simulink subsystem "Motores"  (R2023b)
settings: Solver=VariableStepAuto  StartTime=0.0  StopTime=10.0  RelTol=1e-3
libraries: arduinolib x6, simulink x2
settings Model: Creator=mmgac  LastModifiedBy=jaime
settings OptimizationCC: ReuseModelBlockBuffer=off

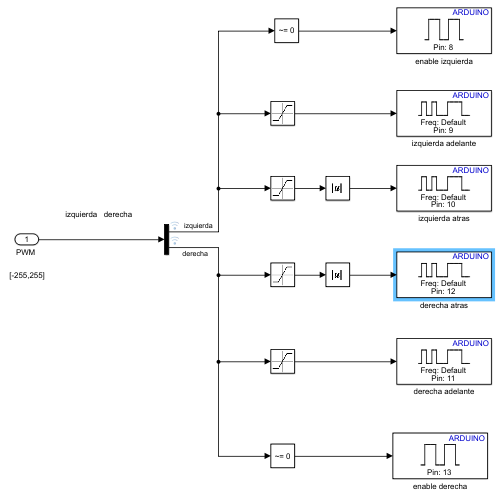
[thumbnail: Simulink's stored preview of the top-level diagram]
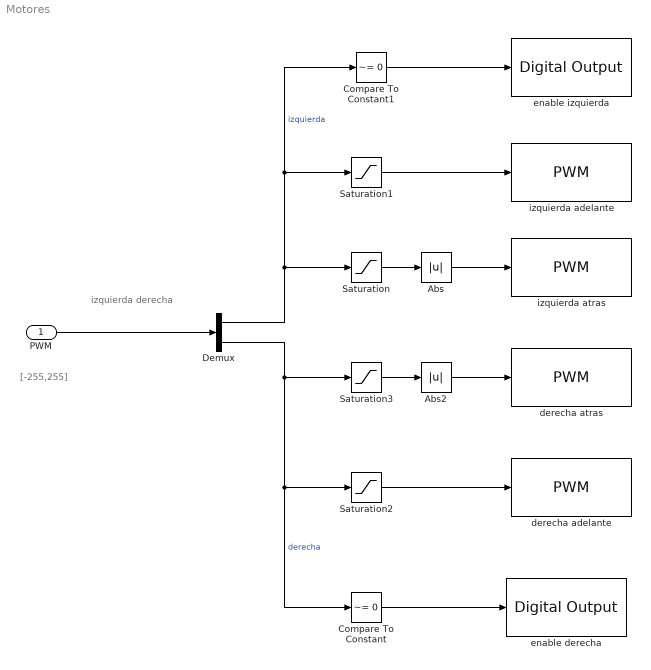
== system Motores ==
  note: izquierda derecha
  note: [-255,255]
  "PWM " : Inport  OutDataTypeStr=int16
  Abs : Abs  OutDataTypeStr=uint8  SaturateOnIntegerOverflow=off
  Abs2 : Abs  OutDataTypeStr=uint8  SaturateOnIntegerOverflow=off
  Compare To Constant : simulink/Logic and Bit Operations/Compare To Constant  relop=~=  const=0  OutDataTypeStr=boolean
  Compare To Constant1 : simulink/Logic and Bit Operations/Compare To Constant  relop=~=  const=0  OutDataTypeStr=boolean
  Demux : Demux  Outputs=2
  Saturation : Saturate  UpperLimit=0  LowerLimit=-255  OutDataTypeStr=int16
  Saturation1 : Saturate  UpperLimit=255  LowerLimit=0  OutDataTypeStr=int16
  Saturation2 : Saturate  UpperLimit=255  LowerLimit=0  OutDataTypeStr=uint16
  Saturation3 : Saturate  UpperLimit=0  LowerLimit=-255  OutDataTypeStr=int16
  derecha adelante : arduinolib/PWM  pinNumber=11  frequencyType=Default  desiredFrequency=490.2  achievableFrequency=490.2
  derecha atras : arduinolib/PWM  pinNumber=12  frequencyType=Default  desiredFrequency=490.2  achievableFrequency=490.2
  enable derecha : arduinolib/Digital Output  pinNumber=13  Direction=output  blockPlatform=arduino
  enable izquierda : arduinolib/Digital Output  pinNumber=8  Direction=output  blockPlatform=arduino
  izquierda adelante : arduinolib/PWM  pinNumber=9  frequencyType=Default  desiredFrequency=490.2  achievableFrequency=490.2
  izquierda atras : arduinolib/PWM  pinNumber=10  frequencyType=Default  desiredFrequency=490.2  achievableFrequency=490.2
  wires:
  Compare To Constant/1 -> enable derecha/1
  Saturation/1 -> Abs/1
  Demux/2 -> Compare To Constant/1, Saturation2/1, Saturation3/1  "derecha"
  Saturation3/1 -> Abs2/1
  Abs/1 -> izquierda atras/1
  Saturation1/1 -> izquierda adelante/1
  Demux/1 -> Compare To Constant1/1, Saturation1/1, Saturation/1  "izquierda"
  Saturation2/1 -> derecha adelante/1
  Abs2/1 -> derecha atras/1
  Compare To Constant1/1 -> enable izquierda/1
  "PWM "/1 -> Demux/1
